simulink model "Read_Sensors"  (R2017a)
settings: Solver=FixedStepDiscrete  StartTime=0.0  StopTime=inf  FixedStep=0.01  RelTol=1e-3  EnableMultiTasking=on
undefined symbols (not defined in the file): HIL
libraries: quarc_library x6
settings Model: SimulationMode=external  ExtModeTrigDuration=1  Creator=drmadill  LastModifiedBy=mbohra
settings SolverCC: PositivePriorityOrder=on
settings DataIOCC: LimitDataPoints=on  SaveFormat=Array  SignalLoggingSaveFormat=ModelDataLogs
settings OptimizationCC: ExpressionDepthLimit=2147483647  LifeSpan=inf
settings DebuggingCC: UnderspecifiedInitializationDetection=Classic  MergeDetectMultiDrivingBlocksExec=none  SolverPrmCheckMsg=warning  FcnCallInpInsideContextMsg=warning  StateNameClashWarn=warning  SFUnexpectedBacktrackingDiag=warning  SFNoUnconditionalDefaultTransitionDiag=warning  SFExecutionAtInitializationDiag=none
settings HardwareCC: ProdBitPerPointer=32  ProdBitPerSizeT=32  ProdBitPerPtrDiffT=32  ProdLargestAtomicFloat=None  ProdIntDivRoundTo=Undefined  ProdEndianess=Unspecified  ProdWordSize=32  ProdHWDeviceType=32-bit Generic
settings ModelReferenceCC: PropagateSignalLabelsOutOfModel=off
settings RTWCC: SystemTargetFile=quarc_linux_duovero_2016.tlc  TemplateMakefile=quarc_linux_duovero_2016_tmf  Description=QUARC Linux DuoVero 2016 Target (QBall 2, QBot 2)
settings STFCustomTargetCC: TargetLibSuffix=.a  TargetPreCompLibLocation=C:\PROGRA~3\QUARC\lib\2017a\LI8355~1\release  ConcurrentExecutionCompliant=on  SystemTargetFile=quarc_linux_duovero_2016.tlc
settings GRTTargetCC: TargetLibSuffix=.a  TargetPreCompLibLocation=C:\PROGRA~3\QUARC\lib\2017a\LI8355~1\release  TargetLangStandard=C89/C90 (ANSI)  ParMdlRefBuildCompliant=off  CompOptLevelCompliant=off  CombineOutputUpdateFcns=off  MatFileLogging=off  CPPClassGenCompliant=off  GRTInterface=on  UseToolchainInfoCompliant=off  ExtMode=on  ExtModeMexFile=quarc_comm  ExtModeMexArgs='-w -d /tmp -uri %u','tcpip://192.168.2.x:17001'
settings ConfigComp: CovMetricSettings=dw  CovHtmlReporting=on  CovSaveCumulativeToWorkspaceVar=on  CovSaveSingleToWorkspaceVar=on  CovExternalEMLEnable=off  CovSFcnEnable=off

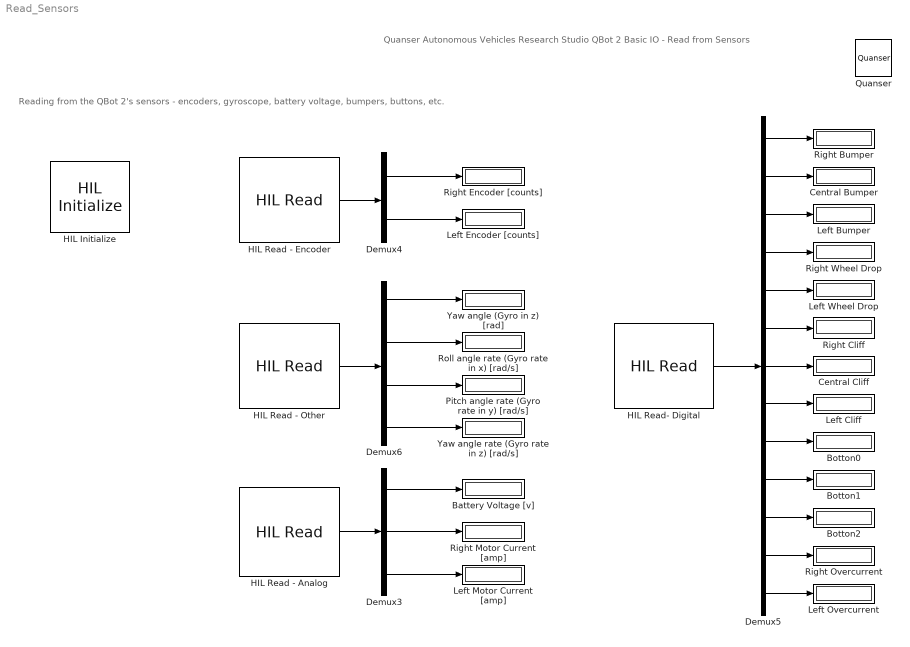
== system Read_Sensors ==
  note: Reading from the QBot 2's sensors - encoders, gyroscope, battery voltage, bumpers, buttons, etc.
  note: Quanser Autonomous Vehicles Research Studio
      | QBot 2 Basic IO - Read from Sensors
  Battery Voltage [v] : Display
      settings: Decimation=20
  Botton0 : Display
      settings: Decimation=20
  Botton1 : Display
      settings: Decimation=20
  Botton2 : Display
      settings: Decimation=20
  Central Bumper : Display
      settings: Decimation=20
  Central Cliff : Display
      settings: Decimation=20
  Demux3 : Demux  Outputs=3
  Demux4 : Demux  Outputs=2
  Demux5 : Demux  Outputs=13
  Demux6 : Demux
  HIL Initialize : quarc_library/Data Acquisition/Generic/Configuration/HIL Initialize  Priority=-99  object_name=HIL-1  board_type=qbot2  board_number=0  board_options=enc0_dir=0;enc0_filter=1;enc0_a=0;enc0_b=0;enc0_z=1;enc0_reload=0;enc1_dir=0;enc1_filter=1;enc1_a=0;enc1_b=0;enc1_z=1;enc1_reload=0;pwm0_immediate=0;pwm1_immediate=0;pwm2_immediate=0;pwm3_immediate=0;  exclusive=off  active=off  hardware_clocks=[]  clock_modes=[]  initial_clock_frequencies=[]  set_clock_params_at_start=off  set_clock_params_at_switch_in=off  set_clock_frequencies_at_start=off  set_clock_frequencies_at_switch_in=off  analog_input_channels=[0:9]  analog_input_configurations=[]  analog_input_maximums=[5 5 5 5 16.5 3.3 3.3 3.3 3.3]  analog_input_minimums=[0 0 0 0 0 0 0 0 0]  set_analog_input_params_at_start=off  set_analog_input_params_at_switch_in=off  analog_output_channels=[]  analog_output_maximums=[]  analog_output_minimums=[]  initial_analog_outputs=[]  final_analog_outputs=[]  watchdog_analog_outputs=[]  set_analog_output_params_at_start=off  set_analog_output_params_at_switch_in=off  set_analog_outputs_at_start=off  set_analog_outputs_at_switch_in=off  set_analog_outputs_at_terminate=off  set_analog_outputs_at_switch_out=off  set_analog_outputs_on_watchdog=off  digital_input_channels=[8:20]  digital_output_channels=[]  digital_output_configuration=[]  initial_digital_outputs=[0]  final_digital_outputs=[0]  watchdog_digital_outputs=[0]  set_digital_output_params_at_start=off  set_digital_output_params_at_switch_in=off  set_digital_outputs_at_start=on  set_digital_outputs_at_switch_in=off  set_digital_outputs_at_terminate=on  set_digital_outputs_at_switch_out=off  set_digital_outputs_on_watchdog=on  encoder_channels=[0:3]  quadrature=[4]  encoder_filter_frequency=[]  initial_encoder_counts=[0]  set_encoder_params_at_start=on  set_encoder_params_at_switch_in=off  set_encoder_counts_at_start=on  set_encoder_counts_at_switch_in=off  pwm_channels=[0:3]  pwm_modes=[0]  pwm_frequency=[20e6/1024]  pwm_configuration=[0]  pwm_alignment=[0]  pwm_polarity=[1]  pwm_leading_deadband=[0]  pwm_trailing_deadband=[0]  initial_pwm_outputs=[0]  final_pwm_outputs=[0]  watchdog_pwm_outputs=[0]  set_pwm_params_at_start=on  set_pwm_params_at_switch_in=off  set_pwm_outputs_at_start=on  set_pwm_outputs_at_switch_in=off  set_pwm_outputs_at_terminate=on  set_pwm_outputs_at_switch_out=off  set_pwm_outputs_on_watchdog=on  other_output_channels=[2000:2001 14000 16000]  initial_other_outputs=[0 0 0 7]  final_other_outputs=[0 0 0 7]  watchdog_other_outputs=[]  set_other_outputs_at_start=on  set_other_outputs_at_switch_in=off  set_other_outputs_at_terminate=on  set_other_outputs_at_switch_out=off  set_other_outputs_on_watchdog=off
  HIL Read - Analog : quarc_library/Data Acquisition/Generic/Immediate I//O/HIL Read  object_name=HIL-1  analog_channels=[4 8 9]  encoder_channels=[]  digital_channels=[]  other_channels=[]  sample_time=qc_get_step_size  active=on  vector_output=on  data_type_mode=Inherit via back propagation  encoder_data_type=double  digital_data_type=boolean
  HIL Read - Encoder : quarc_library/Data Acquisition/Generic/Immediate I//O/HIL Read  object_name=HIL-1  analog_channels=[]  encoder_channels=[2 3]  digital_channels=[]  other_channels=[]  sample_time=qc_get_step_size  active=on  vector_output=on  data_type_mode=Inherit via back propagation  encoder_data_type=double  digital_data_type=boolean
  HIL Read - Other : quarc_library/Data Acquisition/Generic/Immediate I//O/HIL Read  object_name=HIL-1  analog_channels=[]  encoder_channels=[]  digital_channels=[]  other_channels=[1002 3000:3002]  sample_time=qc_get_step_size  active=on  vector_output=on  data_type_mode=Inherit via back propagation  encoder_data_type=double  digital_data_type=boolean
  HIL Read- Digital : quarc_library/Data Acquisition/Generic/Immediate I//O/HIL Read  object_name=HIL-1  analog_channels=[]  encoder_channels=[]  digital_channels=[8:20]  other_channels=[]  sample_time=qc_get_step_size  active=on  vector_output=on  data_type_mode=Inherit via back propagation  encoder_data_type=double  digital_data_type=boolean
  Left Bumper : Display
      settings: Decimation=20
  Left Cliff : Display
      settings: Decimation=20
  Left Encoder [counts] : Display
      settings: Decimation=20
  Left Motor Current [amp] : Display
      settings: Decimation=20
  Left Overcurrent : Display
      settings: Decimation=20
  Left Wheel Drop : Display
      settings: Decimation=20
  Pitch angle rate (Gyro rate in y) [rad/s] : Display
      settings: Decimation=20
  Quanser : quarc_library/Logos/Quanser
  Right Bumper : Display
      settings: Decimation=20
  Right Cliff : Display
      settings: Decimation=20
  Right Encoder [counts] : Display
      settings: Decimation=20
  Right Motor Current [amp] : Display
      settings: Decimation=20
  Right Overcurrent : Display
      settings: Decimation=20
  Right Wheel Drop : Display
      settings: Decimation=20
  Roll angle rate (Gyro rate in x) [rad/s] : Display
      settings: Decimation=20
  Yaw angle (Gyro in z) [rad] : Display
      settings: Decimation=20
  Yaw angle rate (Gyro rate in z) [rad/s] : Display
      settings: Decimation=20
  wires:
  HIL Read - Analog/1 -> Demux3/1
  Demux3/1 -> Battery Voltage [v]/1
  Demux3/2 -> Right Motor Current [amp]/1
  Demux3/3 -> Left Motor Current [amp]/1
  Demux4/1 -> Right Encoder [counts]/1
  Demux4/2 -> Left Encoder [counts]/1
  HIL Read - Encoder/1 -> Demux4/1
  HIL Read- Digital/1 -> Demux5/1
  Demux5/2 -> Central Bumper/1
  Demux5/3 -> Left Bumper/1
  Demux5/4 -> Right Wheel Drop/1
  Demux5/5 -> Left Wheel Drop/1
  Demux5/6 -> Right Cliff/1
  Demux5/7 -> Central Cliff/1
  Demux5/8 -> Left Cliff/1
  Demux5/9 -> Botton0/1
  Demux5/10 -> Botton1/1
  Demux5/11 -> Botton2/1
  Demux5/12 -> Right Overcurrent/1
  Demux5/13 -> Left Overcurrent/1
  HIL Read - Other/1 -> Demux6/1
  Demux6/1 -> Yaw angle (Gyro in z) [rad]/1
  Demux6/2 -> Roll angle rate (Gyro rate in x) [rad/s]/1
  Demux5/1 -> Right Bumper/1
  Demux6/3 -> Pitch angle rate (Gyro rate in y) [rad/s]/1
  Demux6/4 -> Yaw angle rate (Gyro rate in z) [rad/s]/1
